simulink model "Drone2_simulink"  (R2024a)
settings: Solver=ode1be  StartTime=0.0  StopTime=1000  FixedStep=0.001  MaxStep=0.001  MinStep=0.00095  RelTol=1e-3
PreLoadFcn:
  | Drone_data;
model workspace: external: MATLAB File C:\Users\admin\OneDrive - Indian Institute of Technology Jodhpur\IIT JODHPUR\Research Work\Amphibious Drone\MATLAB_CODE\2025\New_Drone\Drone_1\Drone1_simulink_DataFile.m (data not in the file)
undefined symbols (not defined in the file): Environment, Newton, Raphson, Vehicle, X, Y, Z
libraries: sm_lib x1684, nesl_utility x63, slpidlib x25, eeGeneralControl x6, matrix_library x3, rllib x2, simulink x2, fl_lib x1, sharedutil x1, SignalEditorBlockLib x1
(part 1 of 17)
settings Model: Creator=Robotics  LastModifiedBy=Jay Khatri
settings SolverCC: InitialStep=0.00095  MaxConsecutiveMinStep=5  ZeroCrossAlgorithm=Adaptive  EnableFixedStepZeroCrossing=on
settings OptimizationCC: ZeroExternalMemoryAtStartup=off  ZeroInternalMemoryAtStartup=off  InitFltsAndDblsToZero=on
settings DebuggingCC: AlgebraicLoopMsg=none
settings HardwareCC: ProdLongLongMode=on  TargetLongLongMode=on
settings RTWCC: TargetLang=C++  GenerateGPUCode=CUDA
settings GRTTargetCC: TargetLangStandard=C++11 (ISO)  CodeInterfacePackaging=C++ class
settings ExplorerConfigSet: InternalSimMechanicsExplorerSettings="<ExplorerConfiguration><canonicalview>default</canonicalview><AnimationSetting><BasePlaybackSpeed>1.0</BasePlaybackSpeed><PlaybackSpeedFactor>4.0</PlaybackSpeedFactor></AnimationSetting><TilePanel><TileInfo><Tiles Columns=\"1\" Count=\"1\" Rows=\"1\"><Column Weight=\"1\"/><Row Weight=\"1\"/><Tile Height=\"1\" Width=\"1\" X=\"0\" Y=\"0\"/></Tiles></TileInfo><SceneInfo><SceneViewer><BGColor><R>0.60000002384185791</R><G>0.60000002384185791</G><B>0.60000002384185791</B></BGColor><Camera><DoPerspective>on</DoPerspective><Position><X>-30.6897978565157423</X><Y>-15.8041262265084868</Y><Z>-4.45553726878378598</Z></Position><Center><X>-30.1318215683112562</X><Y>-15.047963914826294</Y><Z>-4.79741593175207637</Z></Center><Up><X>0.203078884032637935</X><Y>0.27502726671671418</Y><Z>0.93974409783855084</Z></Up><ViewLimDist>1</ViewLimDist><YLim>0.466307658154998583</YLim><XLim>0.742388726521134967</XLim></Camera></SceneViewer></SceneInfo></TilePanel><MechEditorPanel><Cameras><Camera><Id>Camera1</Id><Value><Name>Camera1</Name><NativeCamera><PositionTrackingFeature>Physical_system.camera.F</PositionTrackingFeature><CenterTrackingFeature>Physical_system.camera.F</CenterTrackingFeature><UpVectorTrackingFeature>Physical_system.camera.F</UpVectorTrackingFeature><CenterTrackingOrigin>off</CenterTrackingOrigin><CenterTrackingDirection>+X</CenterTrackingDirection><UpVectorTrackingDirection>+Z</UpVectorTrackingDirection></NativeCamera></Value></Camera></Cameras><GfxPanelCameraMap><MapElement CameraMLId=\"Camera1\" GfxPanelIndex=\"0\"/></GfxPanelCameraMap><VideoCreator><PlaybackSpeedRatio>8.0</PlaybackSpeedRatio><FrameRate>60</FrameRate><VideoFormat>Motion JPEG AVI</VideoFormat><FrameSize>[1920 1080]</FrameSize></VideoCreator></MechEditorPanel></ExplorerConfiguration>"

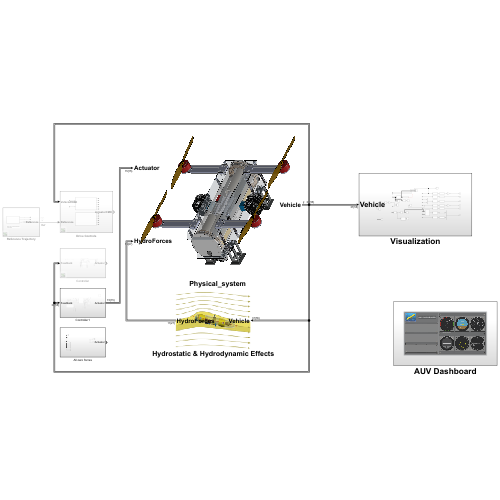
[thumbnail: Simulink's stored preview of the top-level diagram]
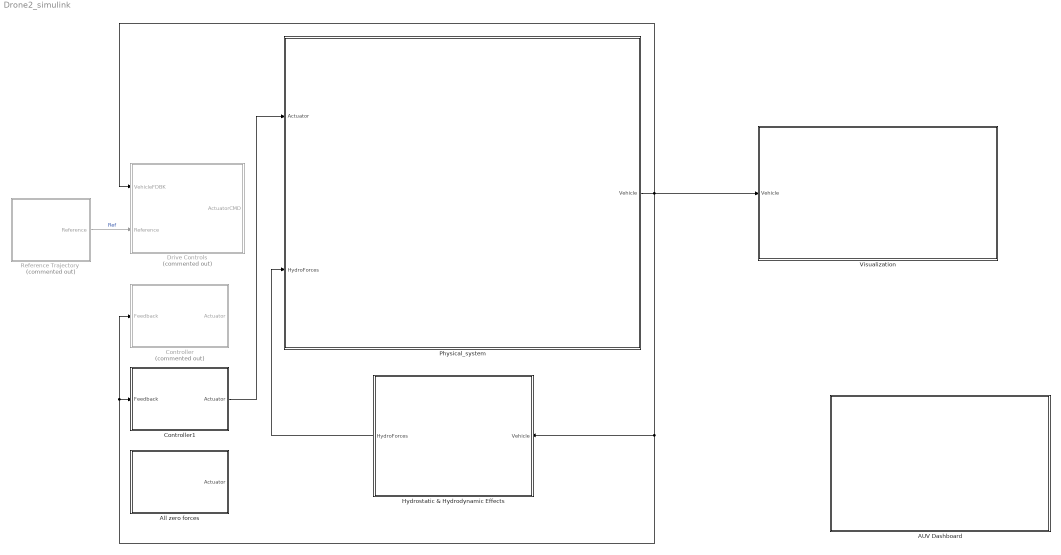
== system Drone2_simulink ==
  AUV Dashboard : Subsystem
  All zero forces : Subsystem
  Controller : Subsystem  Commented=on
  Controller1 : Subsystem
  Drive Controls : Subsystem  Commented=on
  Hydrostatic & Hydrodynamic Effects : Subsystem
      mask Display: image('Drag.png', [0,0,0,0,95,95]);
  Physical_system : Subsystem
      mask Display: image('Drone2_Assembly.PNG');
  Reference Trajectory : Subsystem  Commented=on
  Visualization : Subsystem
  wires:
  Reference Trajectory/1(Reference) -> Drive Controls/2(Reference)  "Ref"
  Physical_system/1(Vehicle) -> Controller/1(Feedback), Controller1/1(Feedback), Hydrostatic & Hydrodynamic Effects/1(Vehicle), Drive Controls/1(VehicleFDBK), Visualization/1(Vehicle)
  Hydrostatic & Hydrodynamic Effects/1(HydroForces) -> Physical_system/2(HydroForces)
  Controller1/1(Actuator) -> Physical_system/1(Actuator)

== system Drone2_simulink/AUV Dashboard ==
  note: AUV DASHBOARD
  note: DEPTH (m)x100
  note: DEPTH (cm)
  note: DEPTH (cm)
  note: SPEED
  note: HEADING
  note: HORIZON
  note: MAIN PROPELLERS (N)
  note: VERTICAL THRUSTERS (N)
  note: HORIZONTAL THRUSTERS (N)
  note: VERTICAL SPEED (ft/min)x10
  note: TURN COORDINATOR
  note: DEPTH (ft)x100
  Airspeed Indicator : AirspeedIndicatorBlock  LabelPosition=Hide  ScaleMin=0  ScaleMax=9
  Altimeter : AltimeterBlock  LabelPosition=Hide
  Artificial Horizon : ArtificialHorizonBlock  LabelPosition=Hide
  Climb Rate Indicator : ClimbIndicatorBlock  LabelPosition=Hide
  Heading Indicator : HeadingIndicatorBlock  LabelPosition=Hide
  Turn Coordinator : TurnCoordinatorBlock  LabelPosition=Hide

== system Drone2_simulink/All zero forces ==
  Constant : Constant  Value=0
  Constant3 : Constant  Value=0
  Constant9 : Constant  Value=0
  Out Bus Element : Outport  PortName=Actuator  Element=Aerial.MotorRB.Thrust
  Out Bus Element1 : Outport  PortName=Actuator  Element=Aerial.MotorRB.Torque
  Out Bus Element2 : Outport  PortName=Actuator  Element=Aerial.MotorRF.Torque
  Out Bus Element5 : Outport  PortName=Actuator  Element=Aerial.MotorRF.Thrust
  Out Bus Element3 : Outport  PortName=Actuator  Element=Aerial.MotorLF.Torque
  Out Bus Element6 : Outport  PortName=Actuator  Element=Aerial.MotorLF.Thrust
  Out Bus Element4 : Outport  PortName=Actuator  Element=Aerial.MotorLB.Torque
  Out Bus Element7 : Outport  PortName=Actuator  Element=Aerial.MotorLB.Thrust
  Out Bus Element8 : Outport  PortName=Actuator  Element=Underwater.ThrusterL.Thrust
  Out Bus Element9 : Outport  PortName=Actuator  Element=Underwater.ThrusterL.Torque
  Out Bus Element10 : Outport  PortName=Actuator  Element=Underwater.ThrusterR.Torque
  Out Bus Element11 : Outport  PortName=Actuator  Element=Underwater.ThrusterR.Thrust
  Out Bus Element12 : Outport  PortName=Actuator  Element=BuoyancyForce.SyringeFL.Force
  Out Bus Element13 : Outport  PortName=Actuator  Element=BuoyancyForce.SyringeFR.Force
  Out Bus Element14 : Outport  PortName=Actuator  Element=BuoyancyForce.SyringeB.Force
  wires:
  Constant/1 -> Out Bus Element9/1, Out Bus Element10/1
  Constant3/1 -> Out Bus Element11/1, Out Bus Element8/1
  Constant9/1 -> Out Bus Element13/1, Out Bus Element12/1, Out Bus Element14/1, Out Bus Element5/1, Out Bus Element2/1, Out Bus Element/1, Out Bus Element1/1, Out Bus Element6/1, Out Bus Element3/1, Out Bus Element7/1, Out Bus Element4/1

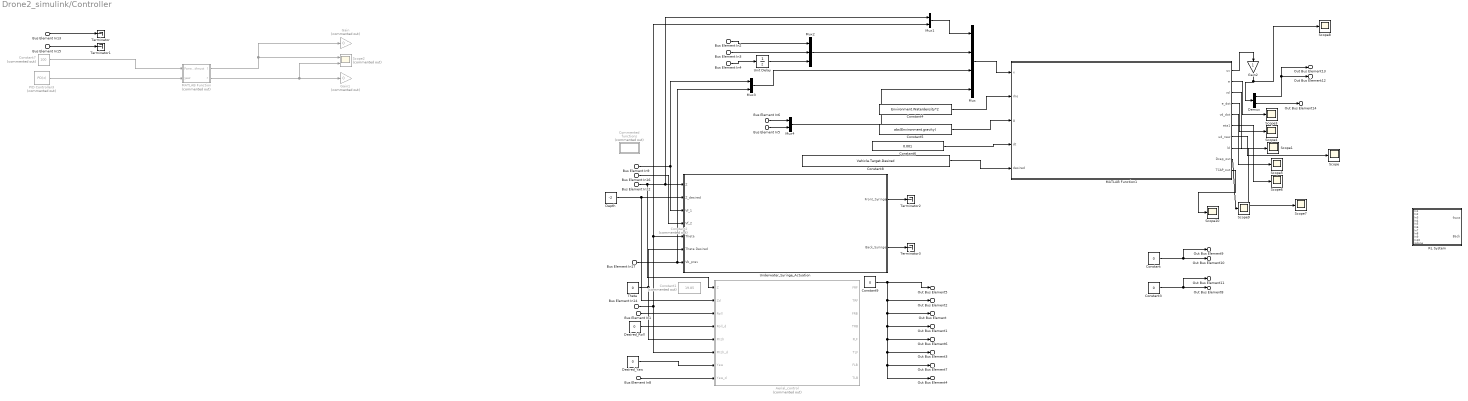
== system Drone2_simulink/Controller ==
  Bus Element In9 : Inport  PortName=Feedback  Element=Buoyancy.Syringe.SyringeFL.Pose
  Bus Element In6 : Inport  PortName=Feedback  Element=Buoyancy.Syringe.SyringeFL.Vel
  Bus Element In16 : Inport  PortName=Feedback  Element=Buoyancy.Syringe.SyringeFR.Pose
  Bus Element In17 : Inport  PortName=Feedback  Element=Buoyancy.Syringe.SyringeB.Pose
  Bus Element In5 : Inport  PortName=Feedback  Element=Buoyancy.Syringe.SyringeB.Vel
  Bus Element In14 : Inport  PortName=Feedback  Element=COM.Derived.Euler.theta
  Bus Element In8 : Inport  PortName=Feedback  Element=COM.Derived.Euler.psi
  Bus Element In1 : Inport  PortName=Feedback  Element=COM.Derived.Euler.phi
  Bus Element In13 : Inport  PortName=Feedback  Element=COM.World.Ve.Vz
  Bus Element In12 : Inport  PortName=Feedback  Element=COM.World.Xe.Z
  Bus Element In15 : Inport  PortName=Feedback  Element=COM.Body.wb.q
  Bus Element In2 : Inport  PortName=Feedback  Element=COM.Body.Vb.u
  Bus Element In3 : Inport  PortName=Feedback  Element=COM.Body.Vb.w
  Bus Element In4 : Inport  PortName=Feedback  Element=COM.Body.dwbdt.qdot
  Aerial_control : Subsystem  Commented=on
  Commented functions : Subsystem  Commented=on
  Constant : Constant  Value=0
  Constant1 : Constant  Commented=on  Value=19.85
  Constant2 : Constant  Commented=on  Value=20
  Constant3 : Constant  Value=0
  Constant4 : Constant  Value=Environment.Waterdensity*2
  Constant5 : Constant  Value=abs(Environment.gravity)
  Constant6 : Constant  Value=0.001
  Constant7 : Constant  Commented=on  Value=100
  Constant8 : Constant  Value=Vehicle.Target.Desired
  Constant9 : Constant  Value=0
  Demux : Demux  Outputs=2
  Depth : Constant  Value=-2
  Desired_Roll : Constant  Value=0
  Desired_Yaw : Constant  Value=0
  Gain : Gain  Commented=on  Gain=0
  Gain1 : Gain  Commented=on  Gain=0
  Gain2 : Gain
  MATLAB Function : MATLAB Function  Commented=on  TreatAsAtomicUnit=on
  MATLAB Function1 : MATLAB Function  TreatAsAtomicUnit=on
  Mux : Mux
  Mux1 : Mux  Inputs=2
  Mux2 : Mux  Inputs=3
  Mux3 : Mux  Inputs=2
  Mux4 : Mux  Inputs=2
  PID Controller3 : slpidlib/PID Controller  Commented=on  Controller=PD  Form=Parallel  TimeDomain=Discrete-time  UseExternalTs=off  SampleTime=0.001  IntegratorMethod=Forward Euler  FilterMethod=Backward Euler  ControllerParametersSource=internal  P=100  I=1  UseKiTs=off  D=5  UseExternalDerivativeSource=off  N=100  UseFilter=on  TunerSelectOption=Transfer Function Based (PID Tuner App)  InitialConditionSource=internal  InitialConditionForIntegrator=0  InitialConditionForFilter=0  DifferentiatorICPrevScaledInput=0  ExternalReset=none  TrackingMode=off  Kt=1  LimitOutput=off  SatLimitsSource=internal  UpperSaturationLimit=inf  LowerSaturationLimit=-inf  LinearizeAsGain=on  AntiWindupMode=none  Kb=1  LimitIntegrator=off  UpperIntegratorSaturationLimit=inf  LowerIntegratorSaturationLimit=-inf  POutMin=[]  POutMax=[]  IOutMin=[]  IOutMax=[]  DOutMin=[]  DOutMax=[]  NOutMin=[]  NOutMax=[]  SumOutMin=[]  SumOutMax=[]  SaturationOutMin=[]  SaturationOutMax=[]  PParamMin=[]  PParamMax=[]  IParamMin=[]  IParamMax=[]  DParamMin=[]  DParamMax=[]  NParamMin=[]  NParamMax=[]  KbParamMin=[]  KbParamMax=[]  KtParamMin=[]  KtParamMax=[]  KbOutMin=[]  KbOutMax=[]  KtOutMin=[]  KtOutMax=[]  IntegratorOutMin=[]  IntegratorOutMax=[]  FilterOutMin=[]  FilterOutMax=[]  SumI1OutMin=[]  SumI1OutMax=[]  SumI2OutMin=[]  SumI2OutMax=[]  SumI3OutMin=[]  SumI3OutMax=[]  SumI4OutMin=[]  SumI4OutMax=[]  SumDOutMin=[]  SumDOutMax=[]  DifferentiatorOutMin=[]  DifferentiatorOutMax=[]  FilterDiffOutCoefMin=[]  FilterDiffOutCoefMax=[]  ReciprocalOutMin=[]  ReciprocalOutMax=[]  SumDenOutMin=[]  SumDenOutMax=[]  SumNumOutMin=[]  SumNumOutMax=[]  DivideOutMin=[]  DivideOutMax=[]  UdiffTsProdOutMin=[]  UdiffTsProdOutMax=[]  NTsProdOutMin=[]  NTsProdOutMax=[]  UintegralTsProdOutMin=[]  UintegralTsProdOutMax=[]  UngainTsProdOutMin=[]  UngainTsProdOutMax=[]  ClampingZeroOutDataTypeStr=Inherit: Inherit via back propagation  ClampingZeroOutMin=[]  ClampingZeroOutMax=[]  FilterDenConstantOutDataTypeStr=Inherit: Inherit via back propagation  FilterDenConstantOutMin=[]  FilterDenConstantOutMax=[]  PCopyOutDataTypeStr=Inherit: Inherit via back propagation  PCopyOutMin=[]  PCopyOutMax=[]  NCopyOutDataTypeStr=Inherit: Inherit via back propagation  NCopyOutMin=[]  NCopyOutMax=[]  IntegratorContinuousStateAttributes=''  IntegratorStateMustResolveToSignalObject=off  IntegratorRTWStateStorageClass=Auto  FilterContinuousStateAttributes=''  FilterStateMustResolveToSignalObject=off  FilterRTWStateStorageClass=Auto  ParallelPVariant=InternalParameters  IdealPVariant=Disabled  IVariant=Disabled  DVariant=InternalParameters  IntegratorVariant=Disabled  SatVariant=Disabled  AWVariant=Disabled  PCopyVariant=Disabled  TRVariant=Disabled  FdbkBlocksVariant=Forward  IdealPFdbkVariant=Disabled  SatFdbkVariant=Disabled  DerivativeFilterVariant=BackwardEulerFilter  NVariant=InternalParameters  NCopyVariant=InternalParameters  FilterICVariant=InternalICsFilter  IntegratorICVariant=Disabled  ExternalResetVariant=Disabled  TRSumVariant=Passthrough  SumFdbkVariant=Disabled  SumVariant=Sum_PD  TsampFilterVariant=InternalTs  TsampNgainVariant=Passthrough  TsampIntegralVariant=Disabled_SignalSpec  ExternalSaturationOutDataTypeStr=Inherit: Same as second input  DerivativeSourceVariant=ErrorSignal
  RL System : Subsystem
  Scope{,1,3..10} (10 alike) : Scope
  Scope2 : Scope  Commented=on  NumInputPorts=2
  Terminator{,1..3} (4 alike) : Terminator
  Theta : Constant  Value=0
  Underwater_Syringe_Actuation : Subsystem
  Unit Delay : UnitDelay  SampleTime=-1  HasFrameUpgradeWarning=on
  Out Bus Element : Outport  PortName=Actuator  Element=Aerial.MotorRB.Thrust
  Out Bus Element1 : Outport  PortName=Actuator  Element=Aerial.MotorRB.Torque
  Out Bus Element2 : Outport  PortName=Actuator  Element=Aerial.MotorRF.Torque
  Out Bus Element5 : Outport  PortName=Actuator  Element=Aerial.MotorRF.Thrust
  Out Bus Element3 : Outport  PortName=Actuator  Element=Aerial.MotorLF.Torque
  Out Bus Element6 : Outport  PortName=Actuator  Element=Aerial.MotorLF.Thrust
  Out Bus Element4 : Outport  PortName=Actuator  Element=Aerial.MotorLB.Torque
  Out Bus Element7 : Outport  PortName=Actuator  Element=Aerial.MotorLB.Thrust
  Out Bus Element8 : Outport  PortName=Actuator  Element=Underwater.ThrusterL.Thrust
  Out Bus Element9 : Outport  PortName=Actuator  Element=Underwater.ThrusterL.Torque
  Out Bus Element10 : Outport  PortName=Actuator  Element=Underwater.ThrusterR.Torque
  Out Bus Element11 : Outport  PortName=Actuator  Element=Underwater.ThrusterR.Thrust
  Out Bus Element12 : Outport  PortName=Actuator  Element=BuoyancyForce.SyringeFL.Force
  Out Bus Element13 : Outport  PortName=Actuator  Element=BuoyancyForce.SyringeFR.Force
  Out Bus Element14 : Outport  PortName=Actuator  Element=BuoyancyForce.SyringeB.Force
  wires:
  Constant3/1 -> Out Bus Element8/1, Out Bus Element11/1
  Bus Element In15/1 -> Terminator1/1
  Bus Element In17/1 -> Mux3/2, Underwater_Syringe_Actuation/7(Vb_prev)
  Constant7/1 -> MATLAB Function/1(Forwardthrust)
  Constant/1 -> Out Bus Element10/1, Out Bus Element9/1
  PID Controller3/1 -> MATLAB Function/2(yaw)
  MATLAB Function/2(r) -> Gain1/1, Scope2/2
  Bus Element In16/1 -> Underwater_Syringe_Actuation/4(Vf_2)
  Bus Element In9/1 -> Mux3/1, Underwater_Syringe_Actuation/3(Vf_1)
  Bus Element In13/1 -> Terminator/1
  Bus Element In12/1 -> Mux1/1, Underwater_Syringe_Actuation/1(Z), Aerial_control/1(Z)
  Depth/1 -> Aerial_control/2(Zd), Underwater_Syringe_Actuation/2(Z_desired)
  Theta/1 -> Underwater_Syringe_Actuation/6(Theta Desired), Aerial_control/5(Pitch)
  Bus Element In14/1 -> Underwater_Syringe_Actuation/5(Theta), Mux1/2, Aerial_control/6(Pitch_d)
  Bus Element In1/1 -> Aerial_control/3(Roll)
  Desired_Roll/1 -> Aerial_control/4(Roll_d)
  Desired_Yaw/1 -> Aerial_control/7(Yaw)
  Bus Element In8/1 -> Aerial_control/8(Yaw_d)
  MATLAB Function/1(l) -> Scope2/1, Gain/1
  Constant9/1 -> Out Bus Element4/1, Out Bus Element7/1, Out Bus Element3/1, Out Bus Element6/1, Out Bus Element1/1, Out Bus Element/1, Out Bus Element2/1, Out Bus Element5/1
  Mux1/1 -> Mux/1
  Bus Element In2/1 -> Mux2/1
  Bus Element In3/1 -> Mux2/2
  Bus Element In4/1 -> Unit Delay/1
  Mux2/1 -> Mux/2
  Bus Element In5/1 -> Mux4/2
  Bus Element In6/1 -> Mux4/1
  Constant4/1 -> MATLAB Function1/2(rho)
  Constant5/1 -> MATLAB Function1/3(g)
  Constant6/1 -> MATLAB Function1/4(dt)
  Constant8/1 -> MATLAB Function1/5(desired)
  MATLAB Function1/1(uc) -> Gain2/1
  Mux/1 -> MATLAB Function1/1(x)
  Mux3/1 -> Mux/3
  Mux4/1 -> Mux/4
  Unit Delay/1 -> Mux2/3
  Underwater_Syringe_Actuation/2(Back_Syringe) -> Terminator3/1
  Underwater_Syringe_Actuation/1(Front_Syringe) -> Terminator2/1
  MATLAB Function1/3(vd) -> Scope1/1
  MATLAB Function1/2(e) -> Scope3/1
  MATLAB Function1/4(e_dot) -> Scope4/1
  MATLAB Function1/5(vd_dot) -> Scope5/1
  MATLAB Function1/6(eta1) -> Scope6/1
  Gain2/1 -> Scope8/1, Demux/1
  Demux/1 -> Out Bus Element13/1, Out Bus Element12/1
  Demux/2 -> Out Bus Element14/1
  MATLAB Function1/8(ld) -> Scope7/1
  MATLAB Function1/7(ud_new) -> Scope/1
  MATLAB Function1/9(Dcap_out) -> Scope9/1
  MATLAB Function1/10(TCAP_out) -> Scope10/1

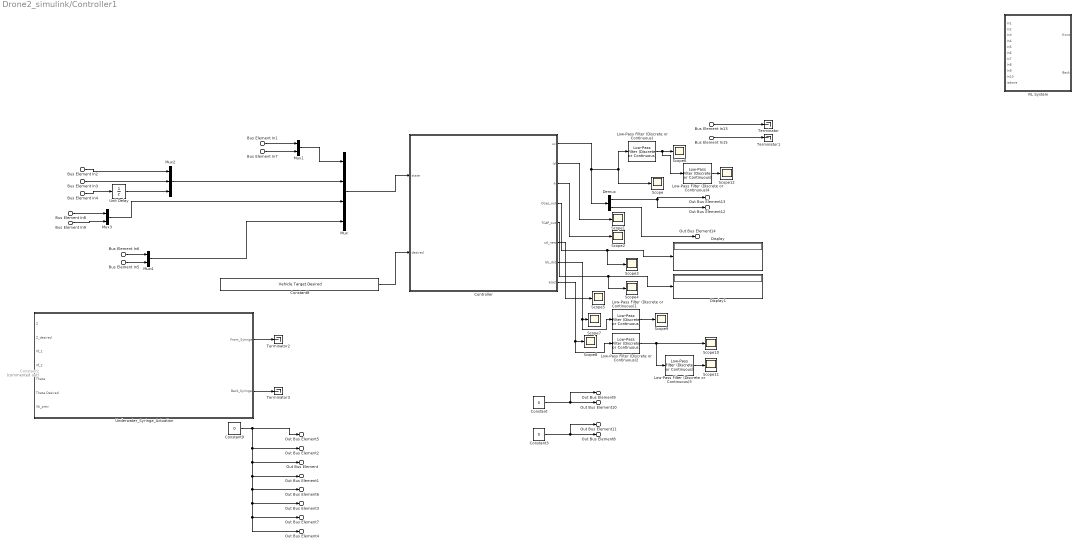
== system Drone2_simulink/Controller1 ==
  Bus Element In6 : Inport  PortName=Feedback  Element=Buoyancy.Syringe.SyringeFL.Vel
  Bus Element In8 : Inport  PortName=Feedback  Element=Buoyancy.Syringe.SyringeFL.Pose
  Bus Element In5 : Inport  PortName=Feedback  Element=Buoyancy.Syringe.SyringeB.Vel
  Bus Element In9 : Inport  PortName=Feedback  Element=Buoyancy.Syringe.SyringeB.Pose
  Bus Element In13 : Inport  PortName=Feedback  Element=COM.World.Ve.Vz
  Bus Element In1 : Inport  PortName=Feedback  Element=COM.World.Xe.Z
  Bus Element In15 : Inport  PortName=Feedback  Element=COM.Body.wb.q
  Bus Element In2 : Inport  PortName=Feedback  Element=COM.Body.Vb.u
  Bus Element In3 : Inport  PortName=Feedback  Element=COM.Body.Vb.w
  Bus Element In4 : Inport  PortName=Feedback  Element=COM.Body.dwbdt.qdot
  Bus Element In7 : Inport  PortName=Feedback  Element=COM.Derived.Euler.theta
  Constant : Constant  Value=0
  Constant2 : Constant  Commented=on  Value=20
  Constant3 : Constant  Value=0
  Constant8 : Constant  Value=Vehicle.Target.Desired
  Constant9 : Constant  Value=0
  Controller : MATLAB Function  TreatAsAtomicUnit=on  mask{m=7.61, IB=diag([0.09331 0.1703 0.2266]), Rsyringe=0.02, l=0.45, RG=[-0.002;0;-0.005], rb=[0;0;0.008], rho=Environment.Waterdensity, g=Environment.gravity, MaxBuoyancyVol=Vehicle.MaxBuoyancyForce/(abs(Environment.gravity*Environment.Waterdensity)), ZS=[0.0273;0.0273;0.0273], Sden=2, dt=0.001, k1e1=1, k1e2=1, k2e1=10, k2e2=100, k2e3=100, k3e1=200, k3e2=200, g1=5, g2=5, g3=0.5, d1=5, d2=5, sigma=6, lb=10*eye(2), MaxIter=10, lambdaLM0=1e-6, tol_r=1e-6, tol_beta=1e-6, minb=0.01, maxb=0.1}
      mask prompts: m "Mass (Kg)"; IB "Inertia Matrix"; Rsyringe "Syringe radius (m)"; l "Length of Vehicle"; RG "Distance of CG from CO"; rb "Distance of CB from CO"; rho "Density"; g "Gravity"; MaxBuoyancyVol "Volume"; ZS "Syringe Z details"; Sden "Syringe Density multiplier"; dt "Sample time"; k1e1 "K11"; k1e2 "K12"; k2e1 "K21"; k2e2 "K22"; k2e3 "K23"; k3e1 "K31"; k3e2 "K32"; g1 "Gamma1"; g2 "Gamma2"; g3 "Gamma3"; d1 "Delta1"; d2 "delta2"; lb "Lambda b"; MaxIter "Max iteration"; lambdaLM0 "Lambda LM0"; tol_r "Relative Tolerance"; tol_beta "Beta tolerance"; minb "Min"; maxb "Max"
  Demux : Demux  Outputs=2
  Display : Display
  Display1 : Display
  Low-Pass Filter (Discrete or Continuous){,1..4} (5 alike) : eeGeneralControl/Low-Pass Filter (Discrete or Continuous)  K=1  T=10  B=inf  A=-inf  init_option=Inherited from block input  x0=0  Ts=-1
  Mux : Mux
  Mux1 : Mux  Inputs=2
  Mux2 : Mux  Inputs=3
  Mux3 : Mux  Inputs=2
  Mux4 : Mux  Inputs=2
  RL System : Subsystem
  Scope{,1..12} (13 alike) : Scope
  Terminator{,1..3} (4 alike) : Terminator
  Underwater_Syringe_Actuation : Subsystem
  Unit Delay : UnitDelay  SampleTime=-1  HasFrameUpgradeWarning=on
  Out Bus Element : Outport  PortName=Actuator  Element=Aerial.MotorRB.Thrust
  Out Bus Element1 : Outport  PortName=Actuator  Element=Aerial.MotorRB.Torque
  Out Bus Element2 : Outport  PortName=Actuator  Element=Aerial.MotorRF.Torque
  Out Bus Element5 : Outport  PortName=Actuator  Element=Aerial.MotorRF.Thrust
  Out Bus Element3 : Outport  PortName=Actuator  Element=Aerial.MotorLF.Torque
  Out Bus Element6 : Outport  PortName=Actuator  Element=Aerial.MotorLF.Thrust
  Out Bus Element4 : Outport  PortName=Actuator  Element=Aerial.MotorLB.Torque
  Out Bus Element7 : Outport  PortName=Actuator  Element=Aerial.MotorLB.Thrust
  Out Bus Element8 : Outport  PortName=Actuator  Element=Underwater.ThrusterL.Thrust
  Out Bus Element9 : Outport  PortName=Actuator  Element=Underwater.ThrusterL.Torque
  Out Bus Element10 : Outport  PortName=Actuator  Element=Underwater.ThrusterR.Torque
  Out Bus Element11 : Outport  PortName=Actuator  Element=Underwater.ThrusterR.Thrust
  Out Bus Element12 : Outport  PortName=Actuator  Element=BuoyancyForce.SyringeFL.Force
  Out Bus Element13 : Outport  PortName=Actuator  Element=BuoyancyForce.SyringeFR.Force
  Out Bus Element14 : Outport  PortName=Actuator  Element=BuoyancyForce.SyringeB.Force
  wires:
  Underwater_Syringe_Actuation/1(Front_Syringe) -> Terminator2/1
  Underwater_Syringe_Actuation/2(Back_Syringe) -> Terminator3/1
  Unit Delay/1 -> Mux2/3
  Mux4/1 -> Mux/4
  Mux3/1 -> Mux/3
  Mux/1 -> Controller/1(state)
  Bus Element In6/1 -> Mux4/1
  Bus Element In5/1 -> Mux4/2
  Mux2/1 -> Mux/2
  Bus Element In4/1 -> Unit Delay/1
  Bus Element In3/1 -> Mux2/2
  Bus Element In2/1 -> Mux2/1
  Mux1/1 -> Mux/1
  Constant9/1 -> Out Bus Element5/1, Out Bus Element2/1, Out Bus Element/1, Out Bus Element1/1, Out Bus Element6/1, Out Bus Element3/1, Out Bus Element7/1, Out Bus Element4/1
  Bus Element In13/1 -> Terminator/1
  Constant/1 -> Out Bus Element9/1, Out Bus Element10/1
  Bus Element In15/1 -> Terminator1/1
  Constant3/1 -> Out Bus Element11/1, Out Bus Element8/1
  Bus Element In1/1 -> Mux1/1
  Bus Element In7/1 -> Mux1/2
  Bus Element In8/1 -> Mux3/1
  Bus Element In9/1 -> Mux3/2
  Constant8/1 -> Controller/2(desired)
  Controller/1(uc) -> Low-Pass Filter (Discrete or Continuous)/1, Scope/1, Demux/1
  Demux/1 -> Out Bus Element12/1, Out Bus Element13/1
  Demux/2 -> Out Bus Element14/1
  Controller/2(ld) -> Scope1/1
  Controller/3(e) -> Scope2/1
  Controller/4(Dcap_out) -> Scope3/1, Display/1
  Controller/5(TCAP_out) -> Scope4/1, Display1/1
  Controller/6(ud_new) -> Scope5/1
  Low-Pass Filter (Discrete or Continuous)/1 -> Low-Pass Filter (Discrete or Continuous)4/1, Scope6/1
  Controller/7(bb_dot) -> Low-Pass Filter (Discrete or Continuous)1/1, Scope7/1
  Low-Pass Filter (Discrete or Continuous)1/1 -> Scope9/1
  Controller/8(eta2) -> Low-Pass Filter (Discrete or Continuous)2/1, Scope8/1
  Low-Pass Filter (Discrete or Continuous)2/1 -> Low-Pass Filter (Discrete or Continuous)3/1, Scope10/1
  Low-Pass Filter (Discrete or Continuous)3/1 -> Scope11/1
  Low-Pass Filter (Discrete or Continuous)4/1 -> Scope12/1

== system Drone2_simulink/Drive Controls ==
  Bus Element In6 : Inport  PortName=VehicleFDBK
  Bus Element In1 : Inport  Port=2  PortName=Reference
  Thrust Controls : Subsystem
  Torque Controls : Subsystem
  Out Bus Element2 : Outport  PortName=ActuatorCMD  Element=Propellers.PPf
  Out Bus Element1 : Outport  PortName=ActuatorCMD  Element=Propellers.PPt
  Out Bus Element4 : Outport  PortName=ActuatorCMD  Element=Propellers.SPf
  Out Bus Element3 : Outport  PortName=ActuatorCMD  Element=Propellers.SPt
  Out Bus Element6 : Outport  PortName=ActuatorCMD  Element=Thrusters.BHTf
  Out Bus Element7 : Outport  PortName=ActuatorCMD  Element=Thrusters.BHTt
  Out Bus Element5 : Outport  PortName=ActuatorCMD  Element=Thrusters.BVTf
  Out Bus Element : Outport  PortName=ActuatorCMD  Element=Thrusters.BVTt
  Out Bus Element8 : Outport  PortName=ActuatorCMD  Element=Thrusters.SHTf
  Out Bus Element9 : Outport  PortName=ActuatorCMD  Element=Thrusters.SHTt
  Out Bus Element10 : Outport  PortName=ActuatorCMD  Element=Thrusters.SVTf
  Out Bus Element11 : Outport  PortName=ActuatorCMD  Element=Thrusters.SVTt
  wires:
  Torque Controls/1(BHTt) -> Out Bus Element7/1
  Torque Controls/2(BVTt) -> Out Bus Element/1
  Torque Controls/3(PPt) -> Out Bus Element1/1
  Torque Controls/4(SPt) -> Out Bus Element3/1
  Torque Controls/5(SHTt) -> Out Bus Element9/1
  Torque Controls/6(SVTt) -> Out Bus Element11/1
  Thrust Controls/3(BVTf) -> Out Bus Element5/1
  Thrust Controls/4(SVTf) -> Out Bus Element10/1
  Thrust Controls/5(BHTf) -> Out Bus Element6/1
  Thrust Controls/6(SHTf) -> Out Bus Element8/1
  Thrust Controls/1(PPf) -> Out Bus Element2/1
  Thrust Controls/2(SPf) -> Out Bus Element4/1
  Bus Element In6/1 -> Thrust Controls/2(VehicleFDBK)
  Bus Element In1/1 -> Thrust Controls/1(Reference)

== system Drone2_simulink/Hydrostatic & Hydrodynamic Effects ==
  Bus Element In6 : Inport  PortName=Vehicle  Element=COM.Body.Vb
  Bus Element In1 : Inport  PortName=Vehicle  Element=COM.Body.wb
  Bus Element In2 : Inport  PortName=Vehicle  Element=COM.Body.dwbdt
  Bus Element In7 : Inport  PortName=Vehicle  Element=COM.World.Xe.Z
  Bus Element In4 : Inport  PortName=Vehicle  Element=COM.World.R
  Bus Element In3 : Inport  PortName=Vehicle  Element=COM.Derived.Body.Abb
  Added Mass Forces : Subsystem
  Buoyancy Force : Subsystem
  Drag Sub system : Subsystem
  Ocean Current : Subsystem
  Wind force : Subsystem
  Bus Element Out3 : Outport  PortName=HydroForces  Element=Drag
  Bus Element Out4 : Outport  PortName=HydroForces  Element=BuoyancyForce
  Bus Element Out1 : Outport  PortName=HydroForces  Element=AddedMass
  Bus Element Out2 : Outport  PortName=HydroForces  Element=OceanCurrentForce
  Bus Element Out5 : Outport  PortName=HydroForces  Element=WindForce
  wires:
  Bus Element In2/1 -> Added Mass Forces/4(dwbdt)
  Bus Element In4/1 -> Wind force/3(Rotation Matrix), Ocean Current/3(Rotation Matrix)
  Bus Element In6/1 -> Ocean Current/1(Vb), Added Mass Forces/1(Vb), Wind force/1(Vb), Drag Sub system/2(Velocity)
  Bus Element In3/1 -> Added Mass Forces/3(Abb)
  Bus Element In7/1 -> Buoyancy Force/1(Z), Ocean Current/2(z), Wind force/2(z), Drag Sub system/1(Altitude)
  Bus Element In1/1 -> Added Mass Forces/2(wb), Drag Sub system/3(Omega_b)
  Drag Sub system/1(Drag) -> Bus Element Out3/1
  Wind force/1(Wind Force) -> Bus Element Out5/1
  Ocean Current/1(OceanCurrent) -> Bus Element Out2/1
  Added Mass Forces/1(AddedMass) -> Bus Element Out1/1
  Buoyancy Force/1(Buoyancy force) -> Bus Element Out4/1

== system Drone2_simulink/Physical_system ==
  Actuator : Inport
  HydroForces : Inport  Port=2
  6-DOF Joint1 : sm_lib/Joints/6-DOF Joint  JointMode=Normal  CompositeWrenchDir=FollowerOnBase  CompositeWrenchFrame=BaseFrame  SenseConstraintForce=off  SenseConstraintTorque=off  SenseTotalForce=off  SenseTotalTorque=off  PxPositionTargetSpecify=on  PxPositionTargetPriority=High  PxPositionTargetValue=Vehicle.InitCond.position(1)  PxPositionTargetValueUnits=m  PxVelocityTargetSpecify=on  PxVelocityTargetPriority=High  PxVelocityTargetValue=Vehicle.InitCond.velocity(1)  PxVelocityTargetValueUnits=m/s  PxEquilibriumPosition=0  PxEquilibriumPositionUnits=m  PxSpringStiffness=0  PxSpringStiffnessUnits=N/m  PxDampingCoefficient=0  PxDampingCoefficientUnits=N/(m/s)  PxLowerLimitSpecify=off  PxLowerLimitBound=-1  PxLowerLimitBoundUnits=m  PxLowerLimitStiffness=1e6  PxLowerLimitStiffnessUnits=N/m  PxLowerLimitDamping=1e3  PxLowerLimitDampingUnits=N/(m/s)  PxLowerLimitTransitionRegionWidth=1e-4  PxLowerLimitTransitionRegionWidthUnits=m  PxUpperLimitSpecify=off  PxUpperLimitBound=1  PxUpperLimitBoundUnits=m  PxUpperLimitStiffness=1e6  PxUpperLimitStiffnessUnits=N/m  PxUpperLimitDamping=1e3  PxUpperLimitDampingUnits=N/(m/s)  PxUpperLimitTransitionRegionWidth=1e-4  PxUpperLimitTransitionRegionWidthUnits=m  PxTorqueActuationMode=NoTorque  PxMotionActuationMode=ComputedMotion  PxSensePosition=off  PxSenseVelocity=off  PxSenseAcceleration=off  PxSenseTorqueForce=off  PxSenseLowerLimitTorqueForce=off  PxSenseUpperLimitTorqueForce=off  PyPositionTargetSpecify=on  PyPositionTargetPriority=High  PyPositionTargetValue=Vehicle.InitCond.position(2)  PyPositionTargetValueUnits=m  PyVelocityTargetSpecify=on  PyVelocityTargetPriority=High  PyVelocityTargetValue=Vehicle.InitCond.velocity(2)  PyVelocityTargetValueUnits=m/s  PyEquilibriumPosition=0  PyEquilibriumPositionUnits=m  PySpringStiffness=0  PySpringStiffnessUnits=N/m  PyDampingCoefficient=0  PyDampingCoefficientUnits=N/(m/s)  PyLowerLimitSpecify=off  PyLowerLimitBound=-1  PyLowerLimitBoundUnits=m  PyLowerLimitStiffness=1e6  PyLowerLimitStiffnessUnits=N/m  PyLowerLimitDamping=1e3  PyLowerLimitDampingUnits=N/(m/s)  PyLowerLimitTransitionRegionWidth=1e-4  PyLowerLimitTransitionRegionWidthUnits=m  PyUpperLimitSpecify=off  PyUpperLimitBound=1  PyUpperLimitBoundUnits=m  PyUpperLimitStiffness=1e6  PyUpperLimitStiffnessUnits=N/m  PyUpperLimitDamping=1e3  PyUpperLimitDampingUnits=N/(m/s)  PyUpperLimitTransitionRegionWidth=1e-4  PyUpperLimitTransitionRegionWidthUnits=m  PyTorqueActuationMode=NoTorque  PyMotionActuationMode=ComputedMotion  PySensePosition=off  PySenseVelocity=off  PySenseAcceleration=off  PySenseTorqueForce=off  PySenseLowerLimitTorqueForce=off  PySenseUpperLimitTorqueForce=off  PzPositionTargetSpecify=on  PzPositionTargetPriority=High  PzPositionTargetValue=Vehicle.InitCond.position(3)  PzPositionTargetValueUnits=m  PzVelocityTargetSpecify=on  PzVelocityTargetPriority=High  PzVelocityTargetValue=Vehicle.InitCond.velocity(3)  PzVelocityTargetValueUnits=m/s  PzEquilibriumPosition=0  PzEquilibriumPositionUnits=m  PzSpringStiffness=0  PzSpringStiffnessUnits=N/m  PzDampingCoefficient=0  PzDampingCoefficientUnits=N/(m/s)  PzLowerLimitSpecify=off  PzLowerLimitBound=-1  PzLowerLimitBoundUnits=m  PzLowerLimitStiffness=1e6  PzLowerLimitStiffnessUnits=N/m  PzLowerLimitDamping=1e3  PzLowerLimitDampingUnits=N/(m/s)  PzLowerLimitTransitionRegionWidth=1e-4  PzLowerLimitTransitionRegionWidthUnits=m  PzUpperLimitSpecify=off  PzUpperLimitBound=1  PzUpperLimitBoundUnits=m  PzUpperLimitStiffness=1e6  PzUpperLimitStiffnessUnits=N/m  PzUpperLimitDamping=1e3  PzUpperLimitDampingUnits=N/(m/s)  PzUpperLimitTransitionRegionWidth=1e-4  PzUpperLimitTransitionRegionWidthUnits=m  PzTorqueActuationMode=NoTorque  PzMotionActuationMode=ComputedMotion  PzSensePosition=off  PzSenseVelocity=off  PzSenseAcceleration=off  PzSenseTorqueForce=off  PzSenseLowerLimitTorqueForce=off  PzSenseUpperLimitTorqueForce=off  SphPositionTargetSpecify=on  SphPositionTargetPriority=High  SphPositionTargetRotationMethod=RotationMatrix  SphPositionTargetFollAlignAxisA=+X  SphPositionTargetBaseAlignAxisA=+Y  SphPositionTargetFollAlignAxisB=+Y  SphPositionTargetBaseAlignAxisB=+Z  SphPositionTargetRotationStandardAxis=+Z  SphPositionTargetRotationAngle=0  SphPositionTargetRotationAngleUnits=deg  SphPositionTargetRotationArbitraryAxis=[0 0 1]  SphPositionTargetRotationSequenceAxes=FollowerAxes  SphPositionTargetRotationSequence=XYX  SphPositionTargetRotationSequenceAngles=[0 0 0]  SphPositionTargetRotationSequenceAnglesUnits=deg  SphPositionTargetRotationMatrix=Vehicle.InitCond.RotMZYX  SphPositionTargetQuaternion=[1 0 0 0]  SphVelocityTargetSpecify=on  SphVelocityTargetPriority=High  SphVelocityTargetValue=Vehicle.InitCond.rotates  SphVelocityTargetValueUnits=deg/s  SphVelocityTargetInFollowerFrame=on  SphEqPosRotationMethod=None  SphEqPosFollAlignAxisA=+X  SphEqPosBaseAlignAxisA=+Y  SphEqPosFollAlignAxisB=+Y  SphEqPosBaseAlignAxisB=+Z  SphEqPosRotationStandardAxis=+Z  SphEqPosRotationAngle=0  SphEqPosRotationAngleUnits=deg  SphEqPosRotationArbitraryAxis=[0 0 1]  SphEqPosRotationSequenceAxes=FollowerAxes  SphEqPosRotationSequence=XYX  SphEqPosRotationSequenceAngles=[0 0 0]  SphEqPosRotationSequenceAnglesUnits=deg  SphEqPosRotationMatrix=[1 0 0;0 1 0;0 0 1]  SphEqPosQuaternion=[1 0 0 0]  SphSpringStiffness=0  SphSpringStiffnessUnits=N*m/deg  SphDampingCoefficient=0  SphDampingCoefficientUnits=N*m/(deg/s)  SphLowerLimitSpecify=off  SphLowerLimitBound=15  SphLowerLimitBoundUnits=deg  SphLowerLimitStiffness=1e4  SphLowerLimitStiffnessUnits=N*m/deg  SphLowerLimitDamping=10  SphLowerLimitDampingUnits=N*m/(deg/s)  SphLowerLimitTransitionRegionWidth=0.1  SphLowerLimitTransitionRegionWidthUnits=deg  SphUpperLimitSpecify=off  SphUpperLimitBound=45  SphUpperLimitBoundUnits=deg  SphUpperLimitStiffness=1e4  SphUpperLimitStiffnessUnits=N*m/deg  SphUpperLimitDamping=10  SphUpperLimitDampingUnits=N*m/(deg/s)  SphUpperLimitTransitionRegionWidth=0.1  SphUpperLimitTransitionRegionWidthUnits=deg  SphTorqueActuationMode=NoTorque  SphActuateTorqueX=off  SphActuateTorqueY=off  SphActuateTorqueZ=off  SphActuateTorque=off  SphActuationFrame=BaseFrame  SphSensePosition=off  SphSenseVelocityX=off  SphSenseVelocityY=off  SphSenseVelocityZ=off  SphSenseVelocity=off  SphSenseAccelerationX=off  SphSenseAccelerationY=off  SphSenseAccelerationZ=off  SphSenseAcceleration=off  SphSenseLowerLimitTorqueMag=off  SphSenseUpperLimitTorqueMag=off  SphSensingFrame=FollowerFrame
  COB_data : Subsystem
      settings: PortSchema="{\"entries\":[{\"content\":{\"sides\":[{\"content\":{\"connectorIds\":[\"LConn1\"]},\"type\":\"ConnectorPlacement.EquallySpacedRectSide\",\"uuid\":\"ce4bd1f6-966c-419e-b3a2-9600ad1f1a9f\"},{\"content\":{\"side\":\"RIGHT\"},\"type\":\"ConnectorPlacement.EquallySpacedRectSide\",\"uuid\":\"b0f91161-b625-4e1f-b78e-415b58b1fabe\"},{\"content\":{\"connectorIds\":[\"LConn2\"],\"side\":\"TOP\"},\"type\":\"ConnectorPlacement.EquallySpacedRectSide\",\"uuid\":\"3d217f50-810e-43e2-bdf0-845eb3b6465a\"},{\"content\":{\"side\":\"BOTTOM\"},\"type\":\"ConnectorPlacement.EquallySpacedRectSide\",\"uuid\":\"49bd3c1b-b520-4a00-93a6-83f0a3b3c3bb\"}]},\"type\":\"ConnectorPlacement.EquallySpacedConnector\",\"uuid\":\"d289346d-dc0f-4cc0-bcd9-c1b77d94d230\"}],\"packageUris\":[\"http://schema.mathworks.com/mf0/Connector/R2020b\"],\"version\":\"1.0\"}"
  COM_Data : Subsystem
      settings: PortSchema="{\"entries\":[{\"content\":{\"sides\":[{\"content\":{\"connectorIds\":[\"LConn1\"]},\"type\":\"ConnectorPlacement.EquallySpacedRectSide\",\"uuid\":\"1e000d2f-58d3-41bb-bd63-01035cb7150c\"},{\"content\":{\"connectorIds\":[\"RConn1\",\"Out1\"],\"side\":\"RIGHT\"},\"type\":\"ConnectorPlacement.EquallySpacedRectSide\",\"uuid\":\"1754a65a-3afe-4d9b-878b-93ac399c3d9d\"},{\"content\":{\"side\":\"TOP\"},\"type\":\"ConnectorPlacement.EquallySpacedRectSide\",\"uuid\":\"1a463dfd-cdd1-494e-b546-7521e6fc03bc\"}]},\"type\":\"ConnectorPlacement.EquallySpacedConnector\",\"uuid\":\"f0725865-f47f-40df-80a9-8598553b9546\"}],\"packageUris\":[\"http://schema.mathworks.com/mf0/Connector/R2020b\"],\"version\":\"1.0\"}"
  Drone_Assembly : Subsystem
      settings: PortSchema="{\"entries\":[{\"content\":{\"sides\":[{\"content\":{\"connectorIds\":[\"In1\",\"LConn1\"]},\"type\":\"ConnectorPlacement.EquallySpacedRectSide\",\"uuid\":\"0540925d-8b88-444e-b03a-b10d9ce31730\"},{\"content\":{\"connectorIds\":[\"Out1\"],\"side\":\"RIGHT\"},\"type\":\"ConnectorPlacement.EquallySpacedRectSide\",\"uuid\":\"3782e599-5bea-4e1a-9d74-9b8e75e09e96\"},{\"content\":{\"connectorIds\":[\"LConn2\"],\"side\":\"TOP\"},\"type\":\"ConnectorPlacement.EquallySpacedRectSide\",\"uuid\":\"7ba90c65-ab86-4cea-9595-ea551b0e3417\"}]},\"type\":\"ConnectorPlacement.EquallySpacedConnector\",\"uuid\":\"3f886a6a-9cba-4f13-9358-882cc77e0e2c\"}],\"packageUris\":[\"http://schema.mathworks.com/mf0/Connector/R2020b\"],\"version\":\"1.0\"}"
      mask Display: image('Drone2_Assembly.PNG');
  Graphic : sm_lib/Body Elements/Graphic  GraphicType=Marker  MarkerShape=Sphere  MarkerSize=10  GraphicVisPropType=SimpleVisualProperties  GraphicDiffuseColor=[0.5 0.5 0.5]  GraphicOpacity=0  GraphicSpecularColor=[0.5 0.5 0.5 1.0]  GraphicAmbientColor=[0.15 0.15 0.15 1.0]  GraphicEmissiveColor=[0.0 0.0 0.0 1.0]  GraphicShininess=75
  Graphic1 : sm_lib/Body Elements/Graphic  GraphicType=Marker  MarkerShape=Sphere  MarkerSize=10  GraphicVisPropType=SimpleVisualProperties  GraphicDiffuseColor=[0.5 0.5 0.5]  GraphicOpacity=0  GraphicSpecularColor=[0.5 0.5 0.5 1.0]  GraphicAmbientColor=[0.15 0.15 0.15 1.0]  GraphicEmissiveColor=[0.0 0.0 0.0 1.0]  GraphicShininess=75
  Hydro Forces & Moments : Subsystem
      settings: PortSchema="{\"entries\":[{\"content\":{\"sides\":[{\"content\":{\"connectorIds\":[\"LConn1\",\"LConn2\"]},\"type\":\"ConnectorPlacement.EquallySpacedRectSide\",\"uuid\":\"9a236f8c-c6e3-4ab2-9fb4-2e996b7f78cc\"},{\"content\":{\"connectorIds\":[\"In1\",\"In2\"],\"side\":\"RIGHT\"},\"type\":\"ConnectorPlacement.EquallySpacedRectSide\",\"uuid\":\"8189b414-8345-4ed6-b1f2-cb1e8295f62f\"},{\"content\":{\"side\":\"TOP\"},\"type\":\"ConnectorPlacement.EquallySpacedRectSide\",\"uuid\":\"7baf8249-5b94-4a82-a7f0-ffd936a54ce9\"}]},\"type\":\"ConnectorPlacement.EquallySpacedConnector\",\"uuid\":\"0b01361b-70c9-4a8a-bc0d-e0750a336c34\"}],\"packageUris\":[\"http://schema.mathworks.com/mf0/Connector/R2020b\"],\"version\":\"1.0\"}"
  Unit Delay : UnitDelay  SampleTime=-1  HasFrameUpgradeWarning=on
  World : Subsystem
  camera : sm_lib/Frames and Transforms/Rigid Transform  RotationMethod=StandardAxis  FollAlignAxisA=+X  BaseAlignAxisA=+Y  FollAlignAxisB=+Y  BaseAlignAxisB=+Z  RotationStandardAxis=+Y  RotationAngle=20  RotationAngleUnits=deg  RotationArbitraryAxis=[0 0 1]  RotationSequenceAxes=FollowerAxes  RotationSequence=XYX  RotationSequenceAngles=[0 0 0]  RotationSequenceAnglesUnits=deg  RotationMatrix=[1 0 0;0 1 0;0 0 1]  Quaternion=[1 0 0 0]  TranslationMethod=Cartesian  TranslationCartesianOffset=[-2 0 1]  TranslationCartesianOffsetUnits=m  TranslationStandardAxis=+Z  TranslationStandardOffset=0  TranslationStandardOffsetUnits=m  TranslationROffset=0  TranslationROffsetUnits=m  TranslationThetaOffset=0  TranslationThetaOffsetUnits=deg  TranslationZOffset=0  TranslationZOffsetUnits=m
  camera1 : sm_lib/Frames and Transforms/Rigid Transform  RotationMethod=None  FollAlignAxisA=+X  BaseAlignAxisA=+Y  FollAlignAxisB=+Y  BaseAlignAxisB=+Z  RotationStandardAxis=+Y  RotationAngle=20  RotationAngleUnits=deg  RotationArbitraryAxis=[0 0 1]  RotationSequenceAxes=FollowerAxes  RotationSequence=XYX  RotationSequenceAngles=[0 0 0]  RotationSequenceAnglesUnits=deg  RotationMatrix=[1 0 0;0 1 0;0 0 1]  Quaternion=[1 0 0 0]  TranslationMethod=Cartesian  TranslationCartesianOffset=Vehicle.InitCond.position +[0 -3 0.25]  TranslationCartesianOffsetUnits=m  TranslationStandardAxis=+Z  TranslationStandardOffset=0  TranslationStandardOffsetUnits=m  TranslationROffset=0  TranslationROffsetUnits=m  TranslationThetaOffset=0  TranslationThetaOffsetUnits=deg  TranslationZOffset=0  TranslationZOffsetUnits=m
  Out Bus Element : Outport  PortName=Vehicle  Element=COM
  Out Bus Element1 : Outport  PortName=Vehicle  Element=Buoyancy
  wires:
  Actuator/1 -> Drone_Assembly/1(Actuator)
  Unit Delay/1 -> Hydro Forces & Moments/2(CenterofMass)
  HydroForces/1 -> Hydro Forces & Moments/1(HydroForces)
  Drone_Assembly/1(buoyancy) -> Out Bus Element1/1
  COM_Data/1(COM) -> Unit Delay/1, Out Bus Element/1
  connections:
  Hydro Forces & Moments/LConn1 -- COM_Data/LConn1 -- camera/LConn1 -- 6-DOF Joint1/RConn1
  Drone_Assembly/LConn2 -- World/RConn2 -- World/RConn1
  Drone_Assembly/LConn1 -- COM_Data/RConn1 -- COB_data/LConn2
  Hydro Forces & Moments/LConn2 -- COB_data/LConn1
  World/RConn3 -- camera1/LConn1 -- 6-DOF Joint1/LConn1
  camera/RConn1 -- Graphic/RConn1
  camera1/RConn1 -- Graphic1/RConn1

== system Drone2_simulink/Reference Trajectory ==
  note: NOTE: Double-click on the Reference Trajectory block to choose the different Active Scenario available.
  Reference Trajectory : SignalEditorBlockLib/Signal Editor  FileName=RefTrajectory.mat  ActiveScenario=StraightDiveNTurn  ActiveSignal=Speed  IsBus=off  OutputBusObjectStr=Bus: BusObject  SampleTime=0  OutputAfterFinalValue=Holding final value  Unit=inherit  PreserveSignalName=on  ApplySigPropsToAllScenarios=on  ApplySigPropsToAllSignals=off
  deg2rad : Gain  Gain=pi/180
  Out Bus Element2 : Outport  PortName=Reference  Element=Speed
  Out Bus Element1 : Outport  PortName=Reference  Element=Depth
  Out Bus Element3 : Outport  PortName=Reference  Element=Heading
  wires:
  Reference Trajectory/1 -> Out Bus Element2/1
  Reference Trajectory/2 -> Out Bus Element1/1
  Reference Trajectory/3 -> deg2rad/1
  deg2rad/1 -> Out Bus Element3/1

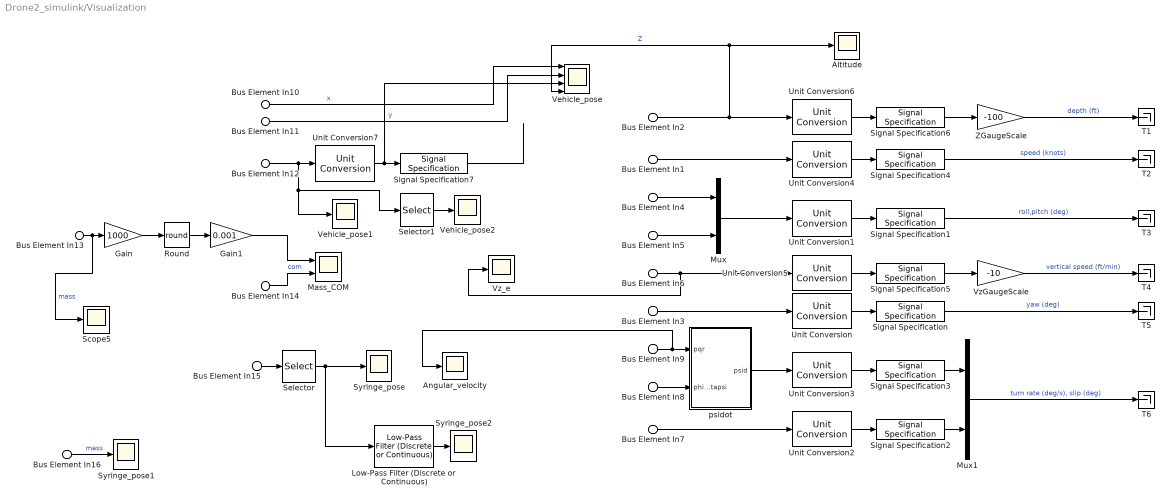
== system Drone2_simulink/Visualization ==
  Bus Element In2 : Inport  PortName=Vehicle  Element=COM.World.Xe.Z
  Bus Element In10 : Inport  PortName=Vehicle  Element=COM.World.Xe.X
  Bus Element In11 : Inport  PortName=Vehicle  Element=COM.World.Xe.Y
  Bus Element In6 : Inport  PortName=Vehicle  Element=COM.World.Ve.Vz
  Bus Element In1 : Inport  PortName=Vehicle  Element=COM.Derived.Body.V
  Bus Element In7 : Inport  PortName=Vehicle  Element=COM.Derived.Body.Incidences.beta
  Bus Element In8 : Inport  PortName=Vehicle  Element=COM.Derived.Euler
  Bus Element In12 : Inport  PortName=Vehicle  Element=COM.Derived.Euler
  Bus Element In3 : Inport  PortName=Vehicle  Element=COM.Derived.Euler.psi
  Bus Element In4 : Inport  PortName=Vehicle  Element=COM.Derived.Euler.phi
  Bus Element In5 : Inport  PortName=Vehicle  Element=COM.Derived.Euler.theta
  Bus Element In9 : Inport  PortName=Vehicle  Element=COM.Body.wb
  Bus Element In13 : Inport  PortName=Vehicle  Element=COM.Body.Mass
  Bus Element In14 : Inport  PortName=Vehicle  Element=COM.Body.COM
  Bus Element In16 : Inport  PortName=Vehicle  Element=COM.Body.Vb
  Bus Element In15 : Inport  PortName=Vehicle  Element=Buoyancy.Syringe
  Altitude : Scope
  Angular_velocity : Scope
  Gain : Gain  Gain=1000
  Gain1 : Gain  Gain=0.001
  Low-Pass Filter (Discrete or Continuous) : eeGeneralControl/Low-Pass Filter (Discrete or Continuous)  K=1  T=10  B=inf  A=-inf  init_option=Inherited from block input  x0=0  Ts=-1
  Mass_COM : Scope  NumInputPorts=2
  Mux : Mux  Inputs=2
  Mux1 : Mux  Inputs=2
  Round : Rounding  Operator=round
  Scope5 : Scope
  Selector : Selector  InputPortWidth=6  IndexOptions=Index vector (dialog)  Indices=[1 3 5]  OutputSizes=1
  Selector1 : Selector  InputPortWidth=3  IndexOptions=Index vector (dialog)  Indices=[2]  OutputSizes=1
  Signal Specification{,1..2,7} (4 alike) : SignalSpecification  Unit=deg
  Signal Specification3 : SignalSpecification  Unit=deg/s
  Signal Specification4 : SignalSpecification  Unit=kn
  Signal Specification5 : SignalSpecification  Unit=ft/min
  Signal Specification6 : SignalSpecification  Unit=ft
  Syringe_pose : Scope
  Syringe_pose1 : Scope
  Syringe_pose2 : Scope
  T{1..6} (6 alike) : Terminator
  Unit Conversion{,1..7} (8 alike) : UnitConversion
  Vehicle_pose : Scope  NumInputPorts=4
  Vehicle_pose1 : Scope
  Vehicle_pose2 : Scope
  VzGaugeScale : Gain  Gain=-10
  Vz_e : Scope
  ZGaugeScale : Gain  Gain=-100
  psidot : Subsystem
  wires:
  Bus Element In2/1 -> Altitude/1, Vehicle_pose/4, Unit Conversion6/1  "Z"
  Bus Element In1/1 -> Unit Conversion4/1
  Unit Conversion4/1 -> Signal Specification4/1
  Bus Element In3/1 -> Unit Conversion/1
  Signal Specification/1 -> T5/1  "yaw (deg)"
  Unit Conversion/1 -> Signal Specification/1
  Bus Element In4/1 -> Mux/1
  Bus Element In5/1 -> Mux/2
  Mux/1 -> Unit Conversion1/1
  Unit Conversion1/1 -> Signal Specification1/1
  Signal Specification1/1 -> T3/1  "roll,pitch (deg)"
  Bus Element In6/1 -> Vz_e/1, Unit Conversion5/1
  Bus Element In7/1 -> Unit Conversion2/1
  Unit Conversion2/1 -> Signal Specification2/1
  Signal Specification2/1 -> Mux1/2
  psidot/1(psid) -> Unit Conversion3/1
  Unit Conversion3/1 -> Signal Specification3/1
  Signal Specification3/1 -> Mux1/1
  Mux1/1 -> T6/1  "turn rate (deg/s), slip (deg)"
  Bus Element In9/1 -> Angular_velocity/1, psidot/1(pqr)
  Bus Element In8/1 -> psidot/2(phithetapsi)
  Signal Specification4/1 -> T2/1  "speed (knots)"
  Unit Conversion5/1 -> Signal Specification5/1
  Signal Specification5/1 -> VzGaugeScale/1
  Unit Conversion6/1 -> Signal Specification6/1
  Signal Specification6/1 -> ZGaugeScale/1
  ZGaugeScale/1 -> T1/1  "depth (ft)"
  VzGaugeScale/1 -> T4/1  "vertical speed (ft/min)"
  Bus Element In10/1 -> Vehicle_pose/1  "x"
  Bus Element In11/1 -> Vehicle_pose/2  "y"
  Bus Element In13/1 -> Scope5/1, Gain/1  "mass"
  Bus Element In14/1 -> Mass_COM/2  "com"
  Bus Element In15/1 -> Selector/1
  Bus Element In12/1 -> Vehicle_pose1/1, Selector1/1, Unit Conversion7/1
  Unit Conversion7/1 -> Vehicle_pose/3, Signal Specification7/1
  Signal Specification7/1 -> ?
  Gain/1 -> Round/1
  Round/1 -> Gain1/1
  Gain1/1 -> Mass_COM/1
  Bus Element In16/1 -> Syringe_pose1/1  "mass"
  Selector/1 -> Low-Pass Filter (Discrete or Continuous)/1, Syringe_pose/1
  Low-Pass Filter (Discrete or Continuous)/1 -> Syringe_pose2/1
  Selector1/1 -> Vehicle_pose2/1
